simulink model "simulink_RPYtoRot_ZXY"  (R2016b)
settings: Solver=VariableStepAuto  StartTime=0.0  StopTime=10.0  RelTol=1e-3
libraries: simulink x5
settings Model: Creator=luminghua  LastModifiedBy=luminghua

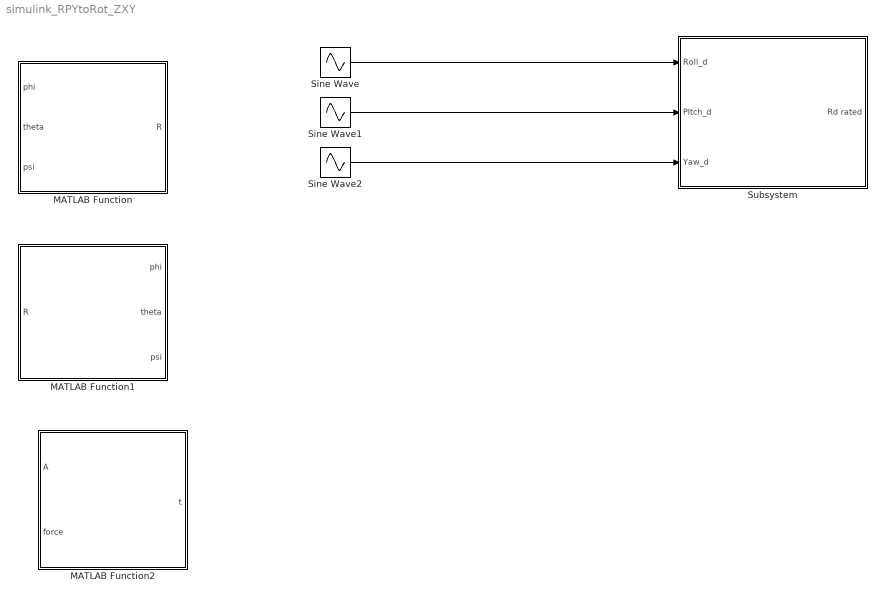
== system simulink_RPYtoRot_ZXY ==
  MATLAB Function : MATLAB Function  TreatAsAtomicUnit=on
  MATLAB Function1 : MATLAB Function  TreatAsAtomicUnit=on
  MATLAB Function2 : MATLAB Function  TreatAsAtomicUnit=on
  Sine Wave : Sin  Amplitude=pi/9  Frequency=pi  SampleTime=0.004
  Sine Wave1 : Sin  Amplitude=pi/9  Frequency=pi  Phase=pi/2  SampleTime=0.004
  Sine Wave2 : Sin  Amplitude=pi/9  Frequency=pi  SampleTime=0.004
  Subsystem : Subsystem
  wires:
  Sine Wave/1 -> Subsystem/1(Roll_d)
  Sine Wave2/1 -> Subsystem/3(Yaw_d)
  Sine Wave1/1 -> Subsystem/2(PItch_d)

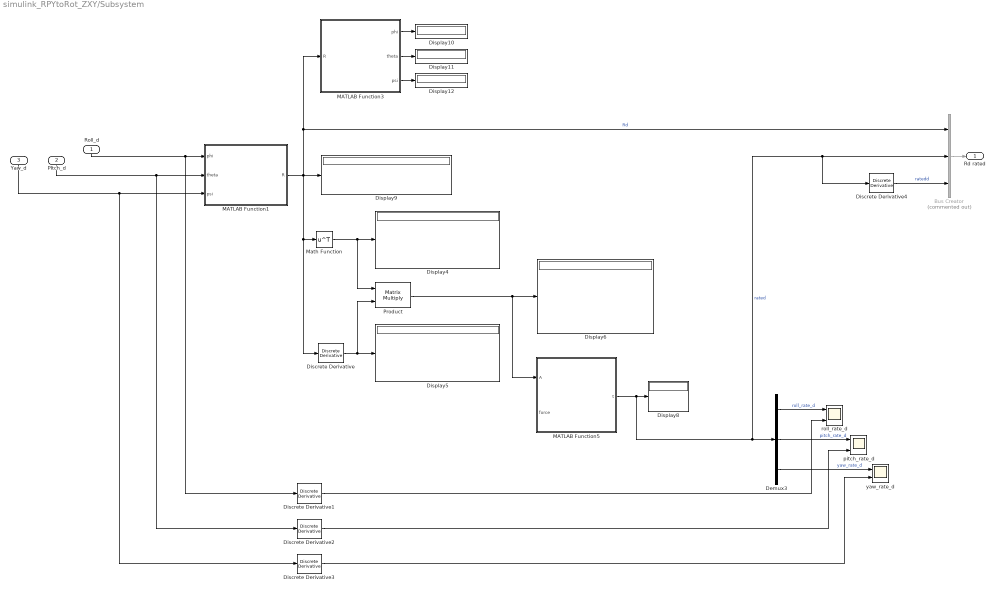
== system simulink_RPYtoRot_ZXY/Subsystem ==
  Roll_d : Inport
  PItch_d : Inport  Port=2
  Yaw_d : Inport  Port=3
  Bus Creator : BusCreator  Commented=on  Inputs=3
  Demux3 : Demux  Outputs=3
  Discrete Derivative{,1..4} (5 alike) : simulink/Discrete/Discrete Derivative  gainval=1.0  ICPrevScaledInput=0.0  OutMin=[]  OutMax=[]  OutDataType=fixdt(1, 16)  OutScaling=2^-10  DoSatur=off
  Display{4..6,8..12} (8 alike) : Display
  MATLAB Function1 : MATLAB Function  TreatAsAtomicUnit=on
  MATLAB Function3 : MATLAB Function  TreatAsAtomicUnit=on
  MATLAB Function5 : MATLAB Function  TreatAsAtomicUnit=on
  Math Function : Math  Operator=transpose  SaturateOnIntegerOverflow=on
  Product : Product  Multiplication=Matrix(*)
  pitch_rate_d : Scope  NumInputPorts=2
  roll_rate_d : Scope  NumInputPorts=2
  yaw_rate_d : Scope  NumInputPorts=2
  Rd rated : Outport
  wires:
  Discrete Derivative3/1 -> yaw_rate_d/2
  MATLAB Function3/2(theta) -> Display11/1
  Discrete Derivative1/1 -> roll_rate_d/2
  Discrete Derivative2/1 -> pitch_rate_d/2
  Product/1 -> MATLAB Function5/1(A), Display6/1
  Discrete Derivative/1 -> Product/2, Display5/1
  MATLAB Function1/1(R) -> MATLAB Function3/1(R), Bus Creator/1, Display9/1, Math Function/1, Discrete Derivative/1  "Rd"
  MATLAB Function3/1(phi) -> Display10/1
  MATLAB Function3/3(psi) -> Display12/1
  Math Function/1 -> Product/1, Display4/1
  MATLAB Function5/1(t) -> Discrete Derivative4/1, Bus Creator/2, Demux3/1, Display8/1  "rated"
  Demux3/3 -> yaw_rate_d/1  "yaw_rate_d"
  Demux3/1 -> roll_rate_d/1  "roll_rate_d"
  Demux3/2 -> pitch_rate_d/1  "pitch_rate_d"
  Roll_d/1 -> Discrete Derivative1/1, MATLAB Function1/1(phi)
  ? -> MATLAB Function5/2(force)
  Yaw_d/1 -> Discrete Derivative3/1, MATLAB Function1/3(psi)
  PItch_d/1 -> Discrete Derivative2/1, MATLAB Function1/2(theta)
  Bus Creator/1 -> Rd rated/1
  Discrete Derivative4/1 -> Bus Creator/3  "ratedd"

== matlab function simulink_RPYtoRot_ZXY/MATLAB Function1 ==
  data: R input; phi output; theta output; psi output
function [phi,theta,psi] = RotToRPY_ZXY(R)
%written by Daniel Mellinger

% 
% R = [ cos(psi)*cos(theta) - sin(phi)*sin(psi)*sin(theta), 
%     cos(theta)*sin(psi) + cos(psi)*sin(phi)*sin(theta), -cos(phi)*sin(theta)]
% 
% [                                 -cos(phi)*sin(psi),
%     cos(phi)*cos(psi),             sin(phi)]
% 
% [ cos(psi)*sin(theta) + cos(theta)*sin(phi)*sin(psi), 
%     sin(psi)*sin(theta) - cos(psi)*cos(theta)*sin(phi),  cos(phi)*cos(theta)]
R = R';
phi = asin(R(2,3));
psi = atan2(-R(2,1)/cos(phi),R(2,2)/cos(phi));
theta = atan2(-R(1,3)/cos(phi),R(3,3)/cos(phi));

== matlab function simulink_RPYtoRot_ZXY/MATLAB Function ==
  data: phi input; R output; theta input; psi input
function R = RPYtoRot_ZXY(phi,theta,psi)
%written by Daniel Mellinger

% BRW = [ cos(psi)*cos(theta) - sin(phi)*sin(psi)*sin(theta), 
%     cos(theta)*sin(psi) + cos(psi)*sin(phi)*sin(theta), -cos(phi)*sin(theta)]
% 
% [                                 -cos(phi)*sin(psi),
%     cos(phi)*cos(psi),             sin(phi)]
% 
% [ cos(psi)*sin(theta) + cos(theta)*sin(phi)*sin(psi), 
%     sin(psi)*sin(theta) - cos(psi)*cos(theta)*sin(phi),
%     cos(phi)*cos(theta)]

R = [ cos(psi)*cos(theta) - sin(phi)*sin(psi)*sin(theta),... 
    cos(theta)*sin(psi) + cos(psi)*sin(phi)*sin(theta), -cos(phi)*sin(theta);...
    -cos(phi)*sin(psi),...
    cos(phi)*cos(psi),             sin(phi);...
    cos(psi)*sin(theta) + cos(theta)*sin(phi)*sin(psi),...
    sin(psi)*sin(theta) - cos(psi)*cos(theta)*sin(phi),...
    cos(phi)*cos(theta)];
    
    R = R';

== matlab function simulink_RPYtoRot_ZXY/MATLAB Function2 ==
  data: A input; t output; force input
function t = vee_map(A, force)
    if(nargin == 1)
        force = false ;
    end
    if(~force)
        if(double(sum(abs(diag(A)))) > 1e-2)
            disp('Error in vee_map() - Nonzero diagonal') ;
%             keyboard ;
        end
    end
    %A = [0 -t(3) t(2) ; t(3) 0 -t(1) ; -t(2) t(1) 0] ;
    t = [A(3,2) ;
         A(1,3) ;
         A(2,1)] ;
end

== matlab function simulink_RPYtoRot_ZXY/Subsystem/MATLAB Function5 ==
  data: A input; t output; force input
function t = vee_map(A, force)
    if(nargin == 1)
        force = false ;
    end
    if(~force)
        if(double(sum(abs(diag(A)))) > 1e-2)
            disp('Error in vee_map() - Nonzero diagonal') ;
%             keyboard ;
        end
    end
    %A = [0 -t(3) t(2) ; t(3) 0 -t(1) ; -t(2) t(1) 0] ;
    t = [A(3,2) ;
         A(1,3) ;
         A(2,1)] ;
end

== matlab function simulink_RPYtoRot_ZXY/Subsystem/MATLAB Function1 ==
  data: phi input; R output; theta input; psi input
function R = RPYtoRot_ZXY(phi,theta,psi)
%written by Daniel Mellinger

% BRW = [ cos(psi)*cos(theta) - sin(phi)*sin(psi)*sin(theta), 
%     cos(theta)*sin(psi) + cos(psi)*sin(phi)*sin(theta), -cos(phi)*sin(theta)]
% 
% [                                 -cos(phi)*sin(psi),
%     cos(phi)*cos(psi),             sin(phi)]
% 
% [ cos(psi)*sin(theta) + cos(theta)*sin(phi)*sin(psi), 
%     sin(psi)*sin(theta) - cos(psi)*cos(theta)*sin(phi),
%     cos(phi)*cos(theta)]

R = [ cos(psi)*cos(theta) - sin(phi)*sin(psi)*sin(theta),... 
    cos(theta)*sin(psi) + cos(psi)*sin(phi)*sin(theta), -cos(phi)*sin(theta);...
    -cos(phi)*sin(psi),...
    cos(phi)*cos(psi),             sin(phi);...
    cos(psi)*sin(theta) + cos(theta)*sin(phi)*sin(psi),...
    sin(psi)*sin(theta) - cos(psi)*cos(theta)*sin(phi),...
    cos(phi)*cos(theta)];
    
    R = R';

== matlab function simulink_RPYtoRot_ZXY/Subsystem/MATLAB Function3 ==
  data: R input; phi output; theta output; psi output
function [phi,theta,psi] = RotToRPY_ZXY(R)
%written by Daniel Mellinger

% 
% R = [ cos(psi)*cos(theta) - sin(phi)*sin(psi)*sin(theta), 
%     cos(theta)*sin(psi) + cos(psi)*sin(phi)*sin(theta), -cos(phi)*sin(theta)]
% 
% [                                 -cos(phi)*sin(psi),
%     cos(phi)*cos(psi),             sin(phi)]
% 
% [ cos(psi)*sin(theta) + cos(theta)*sin(phi)*sin(psi), 
%     sin(psi)*sin(theta) - cos(psi)*cos(theta)*sin(phi),  cos(phi)*cos(theta)]
R = R';
phi = asin(R(2,3));
psi = atan2(-R(2,1)/cos(phi),R(2,2)/cos(phi));
theta = atan2(-R(1,3)/cos(phi),R(3,3)/cos(phi));
